simulink model "ENME562Lab5v2_physical_2018a"  (R2018a)
settings: Solver=ode1  StartTime=0.0  StopTime=20  FixedStep=0.001  RelTol=1e-3  EnableMultiTasking=on
undefined symbols (not defined in the file): HIL
libraries: quarc_library x3, simulink x1
settings Model: SimulationMode=external  ExtModeTrigDuration=10000  Creator=temit  LastModifiedBy=temitope.oni
settings SolverCC: PositivePriorityOrder=on
settings OptimizationCC: LifeSpan=inf
settings RTWCC: SystemTargetFile=quarc_win64.tlc  TemplateMakefile=quarc_default_tmf  Description=QUARC Win64 Target
settings CodeAppCC: StateflowObjectComments=on
settings STFCustomTargetCC: TargetPreCompLibLocation=C:\PROGRA~3\QUARC\lib\2016a\win64\release  TargetLangStandard=C99 (ISO)  ConcurrentExecutionCompliant=on  SystemTargetFile=quarc_win64.tlc
settings GRTTargetCC: TargetPreCompLibLocation=C:\PROGRA~3\QUARC\lib\2018a\win64\release  ParMdlRefBuildCompliant=off  CompOptLevelCompliant=off  CombineOutputUpdateFcns=off  MatFileLogging=off  CPPClassGenCompliant=off  GRTInterface=on  UseToolchainInfoCompliant=off  ExtMode=on  ExtModeMexFile=quarc_comm
settings ConfigComp: CovMetricSettings=dswe

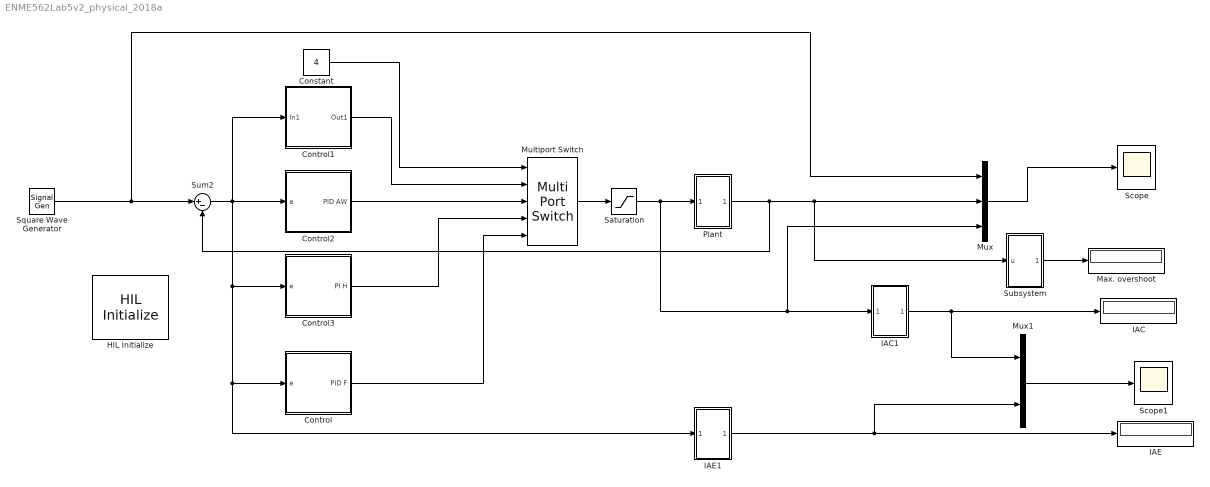
== system ENME562Lab5v2_physical_2018a ==
  Constant : Constant  Value=4
  Control : Subsystem
  Control1 : Subsystem
  Control2 : Subsystem
  Control3 : Subsystem
  HIL Initialize : quarc_library/Data Acquisition/Generic/Configuration/HIL Initialize  object_name=HIL-1  board_type=q8_usb  board_number=0  board_options=update_rate=normal;decimation=1  exclusive=off  active=on  hardware_clocks=[0:2]  clock_modes=[]  initial_clock_frequencies=[]  set_clock_params_at_start=off  set_clock_params_at_switch_in=off  set_clock_frequencies_at_start=off  set_clock_frequencies_at_switch_in=off  analog_input_channels=[0:7]  analog_input_configurations=[]  analog_input_maximums=10  analog_input_minimums=-10  set_analog_input_params_at_start=on  set_analog_input_params_at_switch_in=off  analog_output_channels=[0:7]  analog_output_maximums=10  analog_output_minimums=-10  initial_analog_outputs=[0]  final_analog_outputs=[0]  watchdog_analog_outputs=0  set_analog_output_params_at_start=on  set_analog_output_params_at_switch_in=off  set_analog_outputs_at_start=on  set_analog_outputs_at_switch_in=off  set_analog_outputs_at_terminate=on  set_analog_outputs_at_switch_out=off  set_analog_outputs_on_watchdog=off  digital_input_channels=[]  digital_output_channels=[]  digital_output_configuration=[]  initial_digital_outputs=[1]  final_digital_outputs=[1]  watchdog_digital_outputs=[1]  set_digital_output_params_at_start=off  set_digital_output_params_at_switch_in=off  set_digital_outputs_at_start=on  set_digital_outputs_at_switch_in=off  set_digital_outputs_at_terminate=on  set_digital_outputs_at_switch_out=off  set_digital_outputs_on_watchdog=off  encoder_channels=[0:7]  quadrature=[4]  encoder_filter_frequency=[]  initial_encoder_counts=[0]  set_encoder_params_at_start=on  set_encoder_params_at_switch_in=off  set_encoder_counts_at_start=on  set_encoder_counts_at_switch_in=off  pwm_channels=[0:7]  pwm_modes=0  pwm_frequency=99.532799999999995e6/4095  pwm_configuration=[0]  pwm_alignment=[0]  pwm_polarity=[1]  pwm_leading_deadband=[0]  pwm_trailing_deadband=[0]  initial_pwm_outputs=[0]  final_pwm_outputs=[0]  watchdog_pwm_outputs=[0]  set_pwm_params_at_start=on  set_pwm_params_at_switch_in=off  set_pwm_outputs_at_start=on  set_pwm_outputs_at_switch_in=off  set_pwm_outputs_at_terminate=on  set_pwm_outputs_at_switch_out=off  set_pwm_outputs_on_watchdog=off  other_output_channels=[]  initial_other_outputs=[]  final_other_outputs=[]  watchdog_other_outputs=[]  set_other_outputs_at_start=off  set_other_outputs_at_switch_in=off  set_other_outputs_at_terminate=off  set_other_outputs_at_switch_out=off  set_other_outputs_on_watchdog=off
  IAC : Display
  IAC1 : Subsystem
  IAE : Display
  IAE1 : Subsystem
  Max. overshoot : Display
  Multiport Switch : MultiPortSwitch  Inputs=4
  Mux : Mux  Inputs=3
  Mux1 : Mux  Inputs=2
  Plant : Subsystem
  Saturation : Saturate  UpperLimit=10  LowerLimit=-10
  Scope : Scope
  Scope1 : Scope
  Square Wave Generator : SignalGenerator  WaveForm=square  Amplitude=3  Frequency=0.2
  Subsystem : Subsystem
  Sum2 : Sum  Inputs=|+-
  wires:
  Multiport Switch/1 -> Saturation/1
  IAC1/1(Out1) -> Mux1/1, IAC/1
  Square Wave Generator/1 -> Mux/1, Sum2/1
  Mux/1 -> Scope/1
  Subsystem/1(Out1) -> Max. overshoot/1
  IAE1/1(Out1) -> Mux1/2, IAE/1
  Plant/1(Out1) -> Sum2/2, Subsystem/1(u), Mux/2
  Sum2/1 -> Control1/1(In1), IAE1/1(In1), Control/1(e), Control3/1(e), Control2/1(e)
  Mux1/1 -> Scope1/1
  Control/1(PID F) -> Multiport Switch/5
  Control1/1(Out1) -> Multiport Switch/2
  Control3/1(PI H) -> Multiport Switch/4
  Control2/1(PID AW) -> Multiport Switch/3
  Constant/1 -> Multiport Switch/1
  Saturation/1 -> Plant/1(In1), Mux/3, IAC1/1(In1)

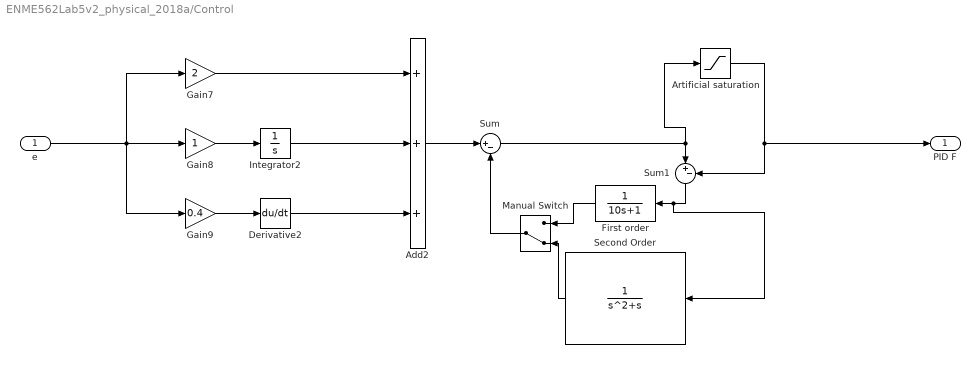
== system ENME562Lab5v2_physical_2018a/Control ==
  e : Inport
  Add2 : Sum  Inputs=+++
  Artificial saturation : Saturate  UpperLimit=10  LowerLimit=-10
  Derivative2 : Derivative
  First order : TransferFcn  Denominator=[10 1]
  Gain7 : Gain  Gain=2
  Gain8 : Gain
  Gain9 : Gain  Gain=0.4
  Integrator2 : Integrator
  Manual Switch : ManualSwitch  CurrentSetting=0
  Second Order : TransferFcn  Denominator=[1 1 0]
  Sum : Sum  Inputs=|+-
  Sum1 : Sum  Inputs=|+-
  PID F : Outport
  wires:
  e/1 -> Gain9/1, Gain8/1, Gain7/1
  Gain7/1 -> Add2/1
  Integrator2/1 -> Add2/2
  Gain8/1 -> Integrator2/1
  Derivative2/1 -> Add2/3
  Gain9/1 -> Derivative2/1
  Artificial saturation/1 -> PID F/1, Sum1/2
  Add2/1 -> Sum/1
  Sum/1 -> Sum1/1, Artificial saturation/1
  Sum1/1 -> Second Order/1, First order/1
  First order/1 -> Manual Switch/1
  Second Order/1 -> Manual Switch/2
  Manual Switch/1 -> Sum/2

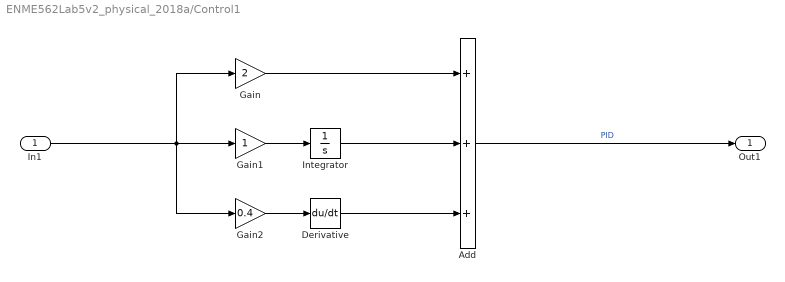
== system ENME562Lab5v2_physical_2018a/Control1 ==
  In1 : Inport
  Add : Sum  Inputs=+++
  Derivative : Derivative
  Gain : Gain  Gain=2
  Gain1 : Gain
  Gain2 : Gain  Gain=0.4
  Integrator : Integrator
  Out1 : Outport  VectorParamsAs1DForOutWhenUnconnected=on
  wires:
  Gain2/1 -> Derivative/1
  Gain/1 -> Add/1
  Derivative/1 -> Add/3
  Integrator/1 -> Add/2
  Gain1/1 -> Integrator/1
  Add/1 -> Out1/1  "PID"
  In1/1 -> Gain2/1, Gain1/1, Gain/1

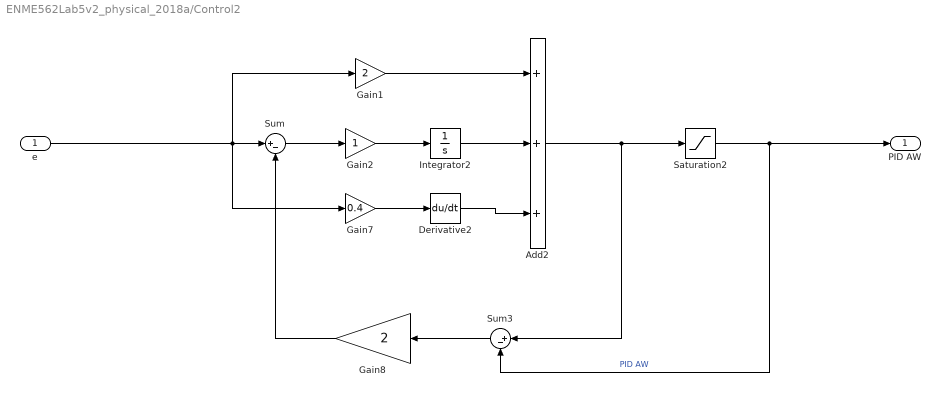
== system ENME562Lab5v2_physical_2018a/Control2 ==
  e : Inport
  Add2 : Sum  Inputs=+++
  Derivative2 : Derivative
  Gain1 : Gain  Gain=2
  Gain2 : Gain
  Gain7 : Gain  Gain=0.4
  Gain8 : Gain  Gain=2
  Integrator2 : Integrator
  Saturation2 : Saturate  UpperLimit=10  LowerLimit=-10
  Sum : Sum  Inputs=|+-
  Sum3 : Sum  Inputs=|+-
  PID AW : Outport
  wires:
  e/1 -> Sum/1, Gain1/1, Gain7/1
  Sum/1 -> Gain2/1
  Integrator2/1 -> Add2/2
  Gain7/1 -> Derivative2/1
  Saturation2/1 -> PID AW/1, Sum3/2  "PID AW"
  Gain2/1 -> Integrator2/1
  Derivative2/1 -> Add2/3
  Gain1/1 -> Add2/1
  Add2/1 -> Sum3/1, Saturation2/1
  Gain8/1 -> Sum/2
  Sum3/1 -> Gain8/1

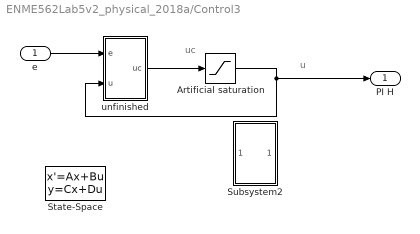
== system ENME562Lab5v2_physical_2018a/Control3 ==
  note: u
  note: uc
  e : Inport
  Artificial saturation : Saturate  UpperLimit=10  LowerLimit=-10
  State-Space : StateSpace  A=-1/2  B=1/2  D=2  InitialCondition=0
  Subsystem2 : Subsystem
  unfinished : Subsystem
  PI H : Outport
  wires:
  Artificial saturation/1 -> unfinished/2(u), PI H/1
  unfinished/1(uc) -> Artificial saturation/1
  e/1 -> unfinished/1(e)

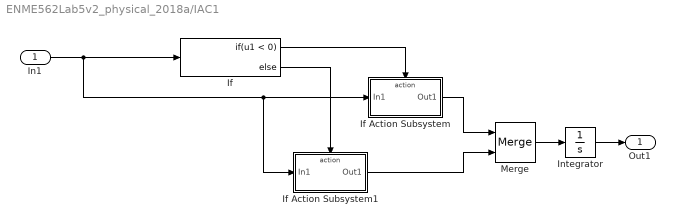
== system ENME562Lab5v2_physical_2018a/IAC1 ==
  In1 : Inport
  If : If  IfExpression=u1 < 0
  If Action Subsystem : Subsystem  TreatAsAtomicUnit=on
  If Action Subsystem1 : Subsystem  TreatAsAtomicUnit=on
  Integrator : Integrator
  Merge : Merge
  Out1 : Outport  VectorParamsAs1DForOutWhenUnconnected=on
  wires:
  If/1 -> If Action Subsystem/Action
  If/2 -> If Action Subsystem1/Action
  In1/1 -> If Action Subsystem1/1(In1), If Action Subsystem/1(In1), If/1
  If Action Subsystem1/1(Out1) -> Merge/2
  Merge/1 -> Integrator/1
  If Action Subsystem/1(Out1) -> Merge/1
  Integrator/1 -> Out1/1

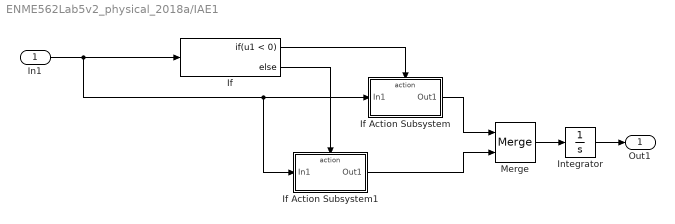
== system ENME562Lab5v2_physical_2018a/IAE1 ==
  In1 : Inport
  If : If  IfExpression=u1 < 0
  If Action Subsystem : Subsystem  TreatAsAtomicUnit=on
  If Action Subsystem1 : Subsystem  TreatAsAtomicUnit=on
  Integrator : Integrator
  Merge : Merge
  Out1 : Outport  VectorParamsAs1DForOutWhenUnconnected=on
  wires:
  Integrator/1 -> Out1/1
  If Action Subsystem/1(Out1) -> Merge/1
  Merge/1 -> Integrator/1
  If Action Subsystem1/1(Out1) -> Merge/2
  In1/1 -> If/1, If Action Subsystem/1(In1), If Action Subsystem1/1(In1)
  If/2 -> If Action Subsystem1/Action
  If/1 -> If Action Subsystem/Action

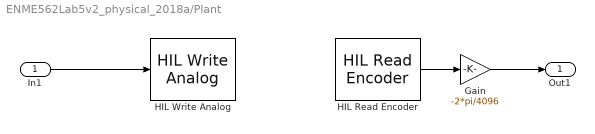
== system ENME562Lab5v2_physical_2018a/Plant ==
  In1 : Inport
  Gain : Gain  Gain=-2*pi/4096
  HIL Read Encoder : quarc_library/Data Acquisition/Generic/Immediate I//O/HIL Read Encoder  object_name=HIL-1  channels=0  sample_time=qc_get_step_size  active=on  vector_output=off  data_type_mode=Inherit via back propagation  data_type=double
  HIL Write Analog : quarc_library/Data Acquisition/Generic/Immediate I//O/HIL Write Analog  object_name=HIL-1  channels=0  sample_time=-1  active=off  vector_input=off
  Out1 : Outport  VectorParamsAs1DForOutWhenUnconnected=on
  wires:
  In1/1 -> HIL Write Analog/1
  HIL Read Encoder/1 -> Gain/1
  Gain/1 -> Out1/1

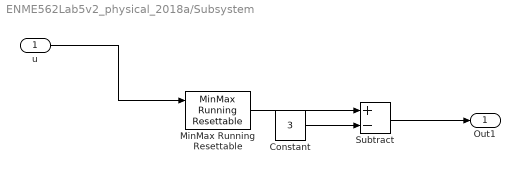
== system ENME562Lab5v2_physical_2018a/Subsystem ==
  u : Inport
  Constant : Constant  Value=3
  MinMax Running Resettable : simulink/Math Operations/MinMax Running Resettable  Function=max  vinit=0.0
  Subtract : Sum  Inputs=+-
  Out1 : Outport  VectorParamsAs1DForOutWhenUnconnected=on
  wires:
  Constant/1 -> Subtract/2
  MinMax Running Resettable/1 -> Subtract/1
  Subtract/1 -> Out1/1
  u/1 -> MinMax Running Resettable/1

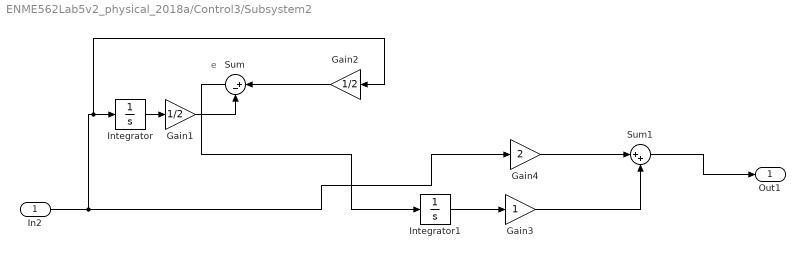
== system ENME562Lab5v2_physical_2018a/Control3/Subsystem2 ==
  note: e
  In2 : Inport
  Gain1 : Gain  Gain=1/2
  Gain2 : Gain  Gain=1/2
  Gain3 : Gain
  Gain4 : Gain  Gain=2
  Integrator : Integrator
  Integrator1 : Integrator
  Sum : Sum  Inputs=|+-
  Sum1 : Sum  Inputs=|++
  Out1 : Outport  VectorParamsAs1DForOutWhenUnconnected=on
  wires:
  Gain2/1 -> Sum/1
  Gain3/1 -> Sum1/2
  In2/1 -> Gain4/1, Gain2/1, Integrator/1
  Integrator1/1 -> Gain3/1
  Gain4/1 -> Sum1/1
  Integrator/1 -> Gain1/1
  Gain1/1 -> Sum/2
  Sum/1 -> Integrator1/1
  Sum1/1 -> Out1/1

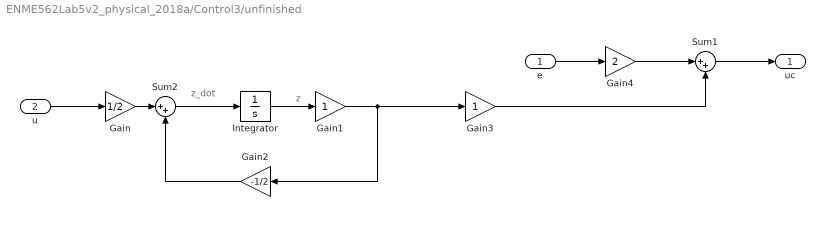
== system ENME562Lab5v2_physical_2018a/Control3/unfinished ==
  note: z_dot
  note: z
  e : Inport
  u : Inport  Port=2
  Gain : Gain  Gain=1/2
  Gain1 : Gain
  Gain2 : Gain  Gain=-1/2
  Gain3 : Gain
  Gain4 : Gain  Gain=2
  Integrator : Integrator
  Sum1 : Sum  Inputs=|++
  Sum2 : Sum  Inputs=|++
  uc : Outport  VectorParamsAs1DForOutWhenUnconnected=on
  wires:
  Gain3/1 -> Sum1/2
  e/1 -> Gain4/1
  Gain1/1 -> Gain2/1, Gain3/1
  Gain4/1 -> Sum1/1
  Integrator/1 -> Gain1/1
  Sum1/1 -> uc/1
  u/1 -> Gain/1
  Gain/1 -> Sum2/1
  Sum2/1 -> Integrator/1
  Gain2/1 -> Sum2/2

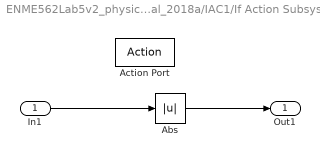
== system ENME562Lab5v2_physical_2018a/IAC1/If Action Subsystem ==
  In1 : Inport
  Action Port : ActionPort  ActionType=then
  Abs : Abs
  Out1 : Outport  VectorParamsAs1DForOutWhenUnconnected=on
  wires:
  In1/1 -> Abs/1
  Abs/1 -> Out1/1

== system ENME562Lab5v2_physical_2018a/IAC1/If Action Subsystem1 ==
  In1 : Inport
  Action Port : ActionPort  ActionType=else
  Out1 : Outport  VectorParamsAs1DForOutWhenUnconnected=on
  wires:
  In1/1 -> Out1/1

== system ENME562Lab5v2_physical_2018a/IAE1/If Action Subsystem ==
  In1 : Inport
  Action Port : ActionPort  ActionType=then
  Abs : Abs
  Out1 : Outport  VectorParamsAs1DForOutWhenUnconnected=on
  wires:
  Abs/1 -> Out1/1
  In1/1 -> Abs/1

== system ENME562Lab5v2_physical_2018a/IAE1/If Action Subsystem1 ==
  In1 : Inport
  Action Port : ActionPort  ActionType=else
  Out1 : Outport  VectorParamsAs1DForOutWhenUnconnected=on
  wires:
  In1/1 -> Out1/1
